simulink model "third_28_02"  (R2024b)
settings: Solver=FixedStepAuto  StartTime=0.0  StopTime=inf  FixedStep=1e-6  MaxStep=1e-4  RelTol=1e-3
values from neighbouring files (symbols this model uses):
  fSW = 10*1000    (= 10000)    [third_28_02_parameters.m]
  l = 10e-3    (= 0.01)    [third_28_02_parameters.m]
  r = 10    [third_28_02_parameters.m]
libraries: simulink x2
settings Model: Creator=Franco  LastModifiedBy=Franco

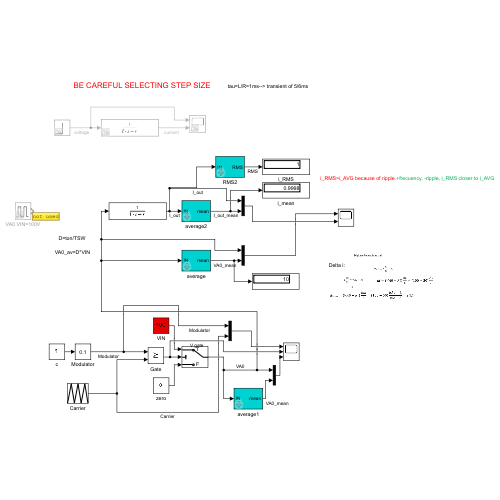
[thumbnail: Simulink's stored preview of the top-level diagram]
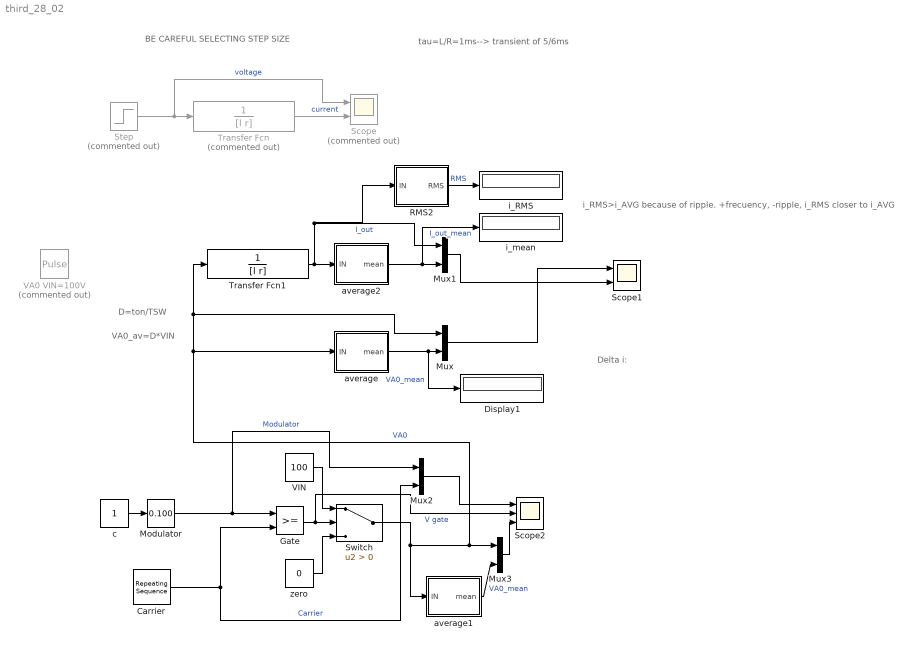
== system third_28_02 ==
  note: i_RMS>i_AVG because of ripple. +frecuency, -ripple, i_RMS closer to i_AVG
  note: Delta i:
  note: BE CAREFUL SELECTING STEP SIZE
  note: VA0_av=D*VIN
  note: D=ton/TSW
  note: tau=L/R=1ms--> transient of 5/6ms
  Carrier : simulink/Sources/Repeating Sequence  rep_seq_t=[0 0.5*(1/fSW) 1*(1/fSW)]  rep_seq_y=[0 1 0]
  Display1 : Display
  Gate : RelationalOperator  OutDataTypeStr=boolean  RndMeth=Simplest  InputSameDT=off
  Modulator : simulink/Math Operations/Slider Gain  gain=0.100  low=0  high=1
  Mux{,1..3} (4 alike) : Mux  Inputs=2
  RMS2 : Subsystem  mask{period=1/fSW}
      mask prompts: period "period [s]"
      mask DialogControl DescTextVar Prompt: calculates the RMS of a periodic function with period specified here
  Scope : Scope  Commented=on  NumInputPorts=2
  Scope1 : Scope  NumInputPorts=2
  Scope2 : Scope  NumInputPorts=3
  Step : Step  Commented=on  After=100  SampleTime=0
  Switch : Switch  Criteria=u2 > Threshold  SaturateOnIntegerOverflow=off  InputSameDT=off
  Transfer Fcn : TransferFcn  Commented=on  Denominator=[l r]
  Transfer Fcn1 : TransferFcn  Denominator=[l r]
  VA0 VIN=100V : DiscretePulseGenerator  Commented=on  PulseType=Time based  Amplitude=100  Period=1/fSW  PulseWidth=50
  VIN : Constant  Value=100
  average : Subsystem  mask{period=1/fSW}
      mask prompts: period "period [s]"
  average1 : Subsystem  mask{period=1/fSW}
      mask prompts: period "period [s]"
  average2 : Subsystem  mask{period=1/fSW}
      mask prompts: period "period [s]"
  c : Constant
  i_RMS : Display
  i_mean : Display
  zero : Constant  Value=0
  wires:
  Step/1 -> Scope/1, Transfer Fcn/1  "voltage"
  Transfer Fcn/1 -> Scope/2  "current"
  average/1(mean) -> Display1/1, Mux/2  "VA0_mean"
  Mux/1 -> Scope1/1
  average2/1(mean) -> i_mean/1, Mux1/2  "I_out_mean"
  Transfer Fcn1/1 -> RMS2/1(IN), Mux1/1, average2/1(IN)  "I_out"
  Mux1/1 -> Scope1/2
  RMS2/1(RMS) -> i_RMS/1  "RMS"
  Carrier/1 -> Gate/2, Mux2/2  "Carrier"
  c/1 -> Modulator/1
  Gate/1 -> Scope2/2, Switch/2  "V gate"
  VIN/1 -> Switch/1
  zero/1 -> Switch/3
  Mux2/1 -> Scope2/1
  Switch/1 -> Transfer Fcn1/1, Mux/1, average/1(IN), Mux3/1, average1/1(IN)  "VA0"
  Modulator/1 -> Mux2/1, Gate/1  "Modulator"
  average1/1(mean) -> Mux3/2  "VA0_mean"
  Mux3/1 -> Scope2/3

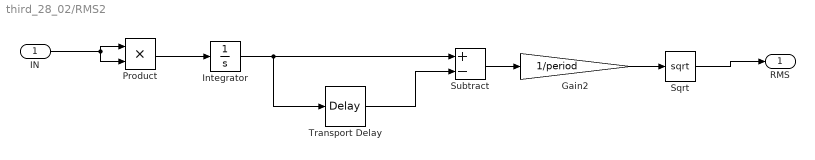
== system third_28_02/RMS2 ==
  IN : Inport
  Gain2 : Gain  Gain=1/period
  Integrator : Integrator
  Product : Product
  Sqrt : Sqrt
  Subtract : Sum  Inputs=+-
  Transport Delay : TransportDelay  DelayTime=period
  RMS : Outport
  wires:
  Sqrt/1 -> RMS/1
  Gain2/1 -> Sqrt/1
  Product/1 -> Integrator/1
  IN/1 -> Product/2, Product/1
  Integrator/1 -> Transport Delay/1, Subtract/1
  Subtract/1 -> Gain2/1
  Transport Delay/1 -> Subtract/2

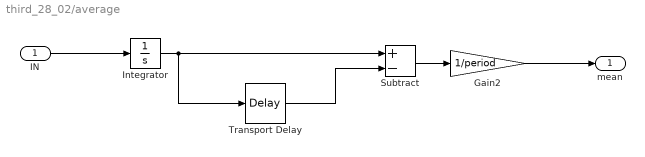
== system third_28_02/average ==
  IN : Inport
  Gain2 : Gain  Gain=1/period
  Integrator : Integrator
  Subtract : Sum  Inputs=+-
  Transport Delay : TransportDelay  DelayTime=period
  mean : Outport
  wires:
  IN/1 -> Integrator/1
  Transport Delay/1 -> Subtract/2
  Subtract/1 -> Gain2/1
  Gain2/1 -> mean/1
  Integrator/1 -> Subtract/1, Transport Delay/1

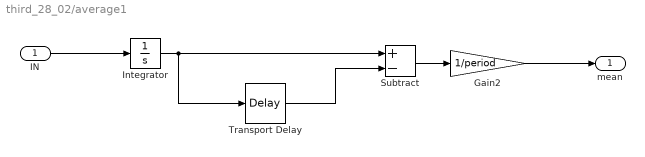
== system third_28_02/average1 ==
  IN : Inport
  Gain2 : Gain  Gain=1/period
  Integrator : Integrator
  Subtract : Sum  Inputs=+-
  Transport Delay : TransportDelay  DelayTime=period
  mean : Outport
  wires:
  Integrator/1 -> Transport Delay/1, Subtract/1
  Gain2/1 -> mean/1
  Subtract/1 -> Gain2/1
  Transport Delay/1 -> Subtract/2
  IN/1 -> Integrator/1

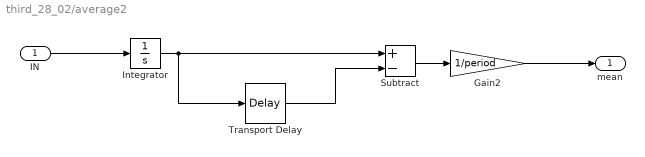
== system third_28_02/average2 ==
  IN : Inport
  Gain2 : Gain  Gain=1/period
  Integrator : Integrator
  Subtract : Sum  Inputs=+-
  Transport Delay : TransportDelay  DelayTime=period
  mean : Outport
  wires:
  Integrator/1 -> Transport Delay/1, Subtract/1
  Gain2/1 -> mean/1
  Subtract/1 -> Gain2/1
  Transport Delay/1 -> Subtract/2
  IN/1 -> Integrator/1
